simulink model "mcb_microchip_pmsm_foc_QDEC_Host_PIC32MK1024MCM"  (R2023b)
settings: Solver=FixedStepDiscrete  StartTime=0.0  StopTime=inf  RelTol=1e-3  EnableMultiTasking=on
values from neighbouring files (symbols this model uses):
  PU_System = mcb_SetPUSystem(pmsm,inverter)    [mcb_microchip_pmsm_foc_QDEC_PIC32MK1024MCF_data.m]
  Ts = T_pwm    (= 8.33333333333e-05)    [mcb_microchip_pmsm_foc_QDEC_PIC32MK1024MCF_data.m]
  Ts_SerialCom = 10*T_pwm    (= 0.000833333333333)    [mcb_microchip_pmsm_foc_QDEC_PIC32MK1024MCF_data.m]
libraries: simulink x6, instrumentseriallib x3
settings Model: Creator=The MathWorks, Inc.  LastModifiedBy=I69995
settings SolverCC: AlgebraicLoopSolver=TrustRegion
settings DataIOCC: LimitDataPoints=on  SaveFormat=Array  ReturnWorkspaceOutputs=off
settings OptimizationCC: LifeSpan=1  EfficientTunableParamExpr=on
settings DebuggingCC: MergeDetectMultiDrivingBlocksExec=none  SolverPrmCheckMsg=warning  ParameterPrecisionLossMsg=none  UnconnectedInputMsg=warning  UnconnectedOutputMsg=warning  UnconnectedLineMsg=warning  AllowSymbolicDim=off  PregeneratedLibrarySubsystemCodeDiagnostic=none  SFUnexpectedBacktrackingDiag=warning  SFNoUnconditionalDefaultTransitionDiag=warning  SFExecutionAtInitializationDiag=none  ArithmeticOperatorsInVariantConditions=warning
settings HardwareCC: ProdBitPerPointer=32  ProdLargestAtomicFloat=None  ProdIntDivRoundTo=Undefined  ProdEndianess=Unspecified  ProdWordSize=32  ProdHWDeviceType=32-bit Generic
settings ModelReferenceCC: EnableRefExpFcnMdlSchedulingChecks=on  PropagateSignalLabelsOutOfModel=off
settings SFSimCC: SimUseLocalCustomCode=off  MATLABDynamicMemAlloc=off
settings RTWCC: Description=Real-Time Workshop Embedded Coder  SystemTargetFile=ert.tlc  TemplateMakefile=ert_default_tmf  GenerateReport=on  RTWUseLocalCustomCode=off  IncludeHyperlinkInReport=on  LaunchReport=on  GenerateTraceInfo=on  GenerateTraceReport=on  GenerateTraceReportSl=on  GenerateTraceReportSf=on  GenerateTraceReportEml=on  DLArmComputeVersion=19.05
settings CodeAppCC: IgnoreCustomStorageClasses=off  StateflowObjectComments=on  InternalIdentifier=Classic
settings ERTTargetCC: MultiwordLength=2048  GenerateSampleERTMain=on  ERTCustomFileTemplate=example_file_process.tlc  ConvertIfToSwitch=off  SuppressUnreachableDefaultCases=off
settings ConfigComp: CovMetricSettings=dw  CovSaveCumulativeToWorkspaceVar=on  CovSaveSingleToWorkspaceVar=on  CovExternalEMLEnable=off  CovSFcnEnable=off

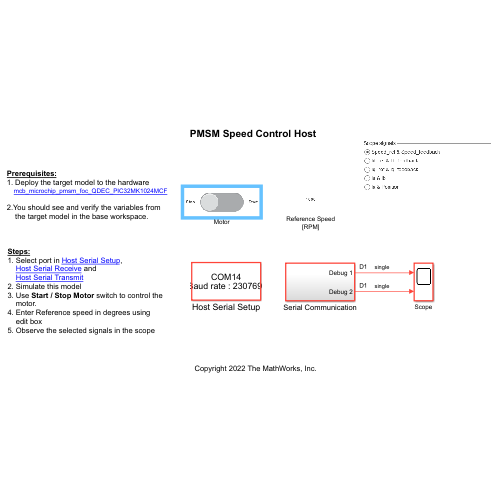
[thumbnail: Simulink's stored preview of the top-level diagram]
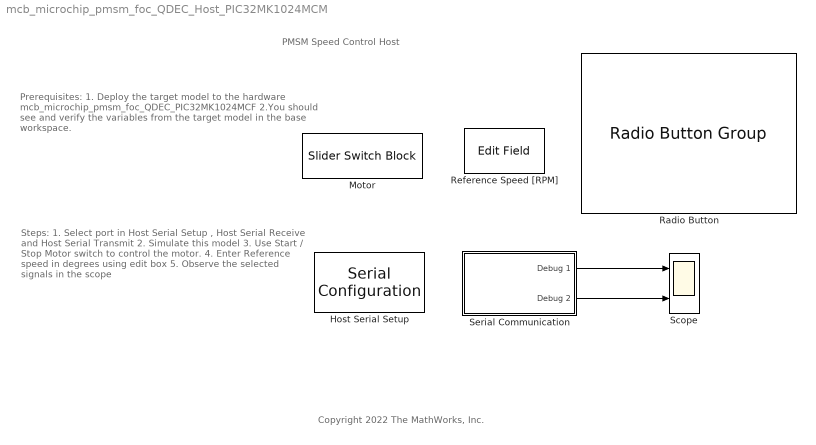
== system mcb_microchip_pmsm_foc_QDEC_Host_PIC32MK1024MCM ==
  note: PMSM Speed Control Host
  note: Copyright 2022 The MathWorks, Inc.
  note: Prerequisites:
      | 1. Deploy the target model to the hardware
      | mcb_microchip_pmsm_foc_QDEC_PIC32MK1024MCF
      |
      | 2.You should see and verify the variables from
      | the target model in the base workspace.
  note: Steps:
      | 1. Select port in Host Serial Setup ,
      | Host Serial Receive and
      | Host Serial Transmit
      | 2. Simulate this model
      | 3. Use Start / Stop Motor switch to control the
      | motor.
      | 4. Enter Reference speed in degrees using
      | edit box
      | 5. Observe the selected signals in the scope
  Host Serial Setup : instrumentseriallib/Serial Configuration  Priority=-99  PortSel=COM14  Port=COM14  ComPort=COM14  BaudRate=2307692  DataBits=8  Parity=none  StopBits=1  ByteOrder=little-endian  FlowControl=none  Timeout=2  SimulateUsing=Interpreted execution  BlockInModel=on  aMode=5
  Motor : SliderSwitchBlock  LabelPosition=Hide
      settings: Values={{'Stop', 'Start'}, [0 1]}
  Radio Button : RadioButtonGroup  LabelPosition=Hide  SelectedLabel=Speed_ref & Speed_feedback  ButtonGroupName=Scope signals
      settings: Values={{'Speed_ref & Speed_feedback', 'Id_ref & Id_feedback', 'Iq_ref & Iq_feedback', 'Ia & Ib', 'Ia & Position'}, [1 2 3 4 5]}
  Reference Speed [RPM] : EditField  LabelPosition=Hide  ShowInitialText=on  Alignment=Center
  Scope : Scope  NumInputPorts=2
  Serial Communication : Subsystem
  wires:
  Serial Communication/1(Debug 1) -> Scope/1
  Serial Communication/2(Debug 2) -> Scope/2

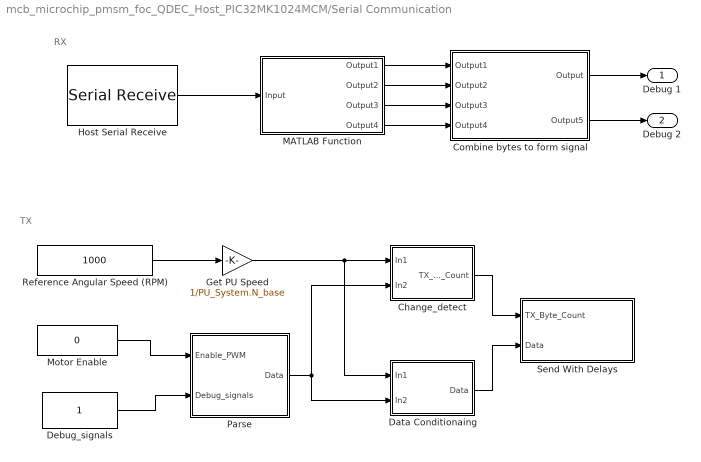
== system mcb_microchip_pmsm_foc_QDEC_Host_PIC32MK1024MCM/Serial Communication ==
  note: RX
  note: TX
  Change_detect : Subsystem
  Combine bytes to form signal : Subsystem
  Data Conditionaing : Subsystem  VariantControl=~isequal(dataType, 'single')
  Debug_signals : Constant  OutDataTypeStr=uint8  SampleTime=600 * Ts
  Get PU Speed : Gain  Gain=1/PU_System.N_base  OutDataTypeStr=fixdt(1,16,10)  RndMeth=Simplest
  Host Serial Receive : instrumentseriallib/Serial Receive  PortSel=COM14  Port=COM14  ComPort=COM14  DataType=uint8  SaveDataType=uint8  ToggleHeader=on  Header='S'  ToggleTerminator=on  Terminator=Custom terminator  CustomTerminator='E'  InputFormat=Row major  ToggleDataSize=on  DataSize=[60 4]  EnableBlockingMode=on  ActionDataUnavailable=Output last received value  ActionWhenDataUnavailable=Output last received value  CustomValue=15  SampleTime=60 * Ts_SerialCom  SimulateUsing=Interpreted execution  BlockInModel=on  aMode=5
  MATLAB Function : MATLAB Function  TreatAsAtomicUnit=on
  Motor Enable : Constant  Value=0  VectorParams1D=off  OutDataTypeStr=uint8  SampleTime=600 * Ts
  Parse : Subsystem
  Reference Angular Speed (RPM) : Constant  Value=1000  VectorParams1D=off  OutDataTypeStr=single  SampleTime=600 * Ts
  Send With Delays : Subsystem
  Debug 1 : Outport
  Debug 2 : Outport  Port=2
  wires:
  Host Serial Receive/1 -> MATLAB Function/1(Input)
  Combine bytes to form signal/1(Output) -> Debug 1/1
  Combine bytes to form signal/2(Output5) -> Debug 2/1
  Debug_signals/1 -> Parse/2(Debug_signals)
  Motor Enable/1 -> Parse/1(Enable_PWM)
  Parse/1(Data) -> Data Conditionaing/2(In2), Change_detect/2(In2)
  Reference Angular Speed (RPM)/1 -> Get PU Speed/1
  MATLAB Function/1(Output1) -> Combine bytes to form signal/1(Output1)
  MATLAB Function/2(Output2) -> Combine bytes to form signal/2(Output2)
  MATLAB Function/3(Output3) -> Combine bytes to form signal/3(Output3)
  MATLAB Function/4(Output4) -> Combine bytes to form signal/4(Output4)
  Change_detect/1(TX_Byte_Count) -> Send With Delays/1(TX_Byte_Count)
  Data Conditionaing/1(Data) -> Send With Delays/2(Data)
  Get PU Speed/1 -> Data Conditionaing/1(In1), Change_detect/1(In1)

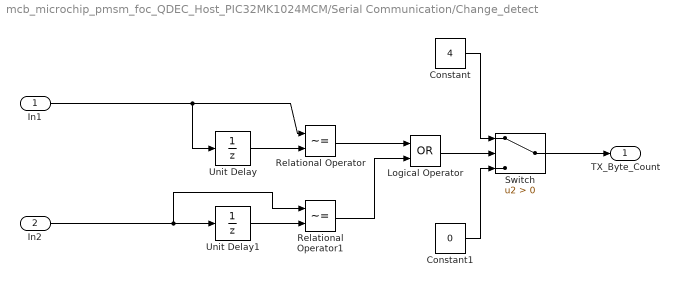
== system mcb_microchip_pmsm_foc_QDEC_Host_PIC32MK1024MCM/Serial Communication/Change_detect ==
  In1 : Inport
  In2 : Inport  Port=2
  Constant : Constant  Value=4  OutDataTypeStr=uint8
  Constant1 : Constant  Value=0  OutDataTypeStr=uint8
  Logical Operator : Logic  Operator=OR  AllPortsSameDT=off  OutDataTypeStr=boolean
  Relational Operator : RelationalOperator  Operator=~=  OutDataTypeStr=boolean  InputSameDT=off
  Relational Operator1 : RelationalOperator  Operator=~=  OutDataTypeStr=boolean  InputSameDT=off
  Switch : Switch  Criteria=u2 > Threshold  SaturateOnIntegerOverflow=off  InputSameDT=off
  Unit Delay : UnitDelay  InitialCondition=0.5  SampleTime=-1  HasFrameUpgradeWarning=on
  Unit Delay1 : UnitDelay  SampleTime=-1  HasFrameUpgradeWarning=on
  TX_Byte_Count : Outport  VectorParamsAs1DForOutWhenUnconnected=off
  wires:
  Relational Operator/1 -> Logical Operator/1
  In1/1 -> Relational Operator/1, Unit Delay/1
  Unit Delay/1 -> Relational Operator/2
  Unit Delay1/1 -> Relational Operator1/2
  Relational Operator1/1 -> Logical Operator/2
  In2/1 -> Unit Delay1/1, Relational Operator1/1
  Constant1/1 -> Switch/3
  Constant/1 -> Switch/1
  Logical Operator/1 -> Switch/2
  Switch/1 -> TX_Byte_Count/1

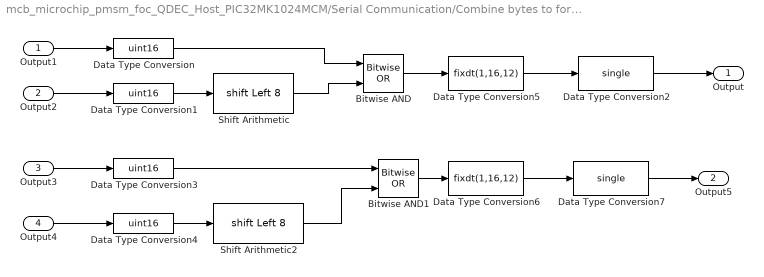
== system mcb_microchip_pmsm_foc_QDEC_Host_PIC32MK1024MCM/Serial Communication/Combine bytes to form signal ==
  Output1 : Inport
  Output2 : Inport  Port=2
  Output3 : Inport  Port=3
  Output4 : Inport  Port=4
  Bitwise AND : simulink/Logic and Bit Operations/Bitwise Operator  logicop=OR  UseBitMask=off  NumInputPorts=2  BitMask=bin2dec('11011001')  BitMaskRealWorld=Stored Integer
  Bitwise AND1 : simulink/Logic and Bit Operations/Bitwise Operator  logicop=OR  UseBitMask=off  NumInputPorts=2  BitMask=bin2dec('11011001')  BitMaskRealWorld=Stored Integer
  Data Type Conversion{,1,3..4} (4 alike) : DataTypeConversion  OutDataTypeStr=uint16  RndMeth=Simplest  SaturateOnIntegerOverflow=off
  Data Type Conversion2 : DataTypeConversion  OutDataTypeStr=single  RndMeth=Simplest  SaturateOnIntegerOverflow=off
  Data Type Conversion5 : DataTypeConversion  OutDataTypeStr=fixdt(1,16,12)  ConvertRealWorld=Stored Integer (SI)  RndMeth=Simplest  SaturateOnIntegerOverflow=off
  Data Type Conversion6 : DataTypeConversion  OutDataTypeStr=fixdt(1,16,12)  ConvertRealWorld=Stored Integer (SI)  RndMeth=Simplest  SaturateOnIntegerOverflow=off
  Data Type Conversion7 : DataTypeConversion  OutDataTypeStr=single  RndMeth=Simplest  SaturateOnIntegerOverflow=off
  Shift Arithmetic : ArithShift  BitShiftNumber=8  BitShiftDirection=Left
  Shift Arithmetic2 : ArithShift  BitShiftNumber=8  BitShiftDirection=Left
  Output : Outport
  Output5 : Outport  Port=2
  wires:
  Output1/1 -> Data Type Conversion/1
  Data Type Conversion5/1 -> Data Type Conversion2/1
  Output2/1 -> Data Type Conversion1/1
  Bitwise AND/1 -> Data Type Conversion5/1
  Data Type Conversion1/1 -> Shift Arithmetic/1
  Data Type Conversion/1 -> Bitwise AND/1
  Output3/1 -> Data Type Conversion3/1
  Output4/1 -> Data Type Conversion4/1
  Data Type Conversion4/1 -> Shift Arithmetic2/1
  Shift Arithmetic/1 -> Bitwise AND/2
  Bitwise AND1/1 -> Data Type Conversion6/1
  Data Type Conversion6/1 -> Data Type Conversion7/1
  Data Type Conversion3/1 -> Bitwise AND1/1
  Shift Arithmetic2/1 -> Bitwise AND1/2
  Data Type Conversion2/1 -> Output/1
  Data Type Conversion7/1 -> Output5/1

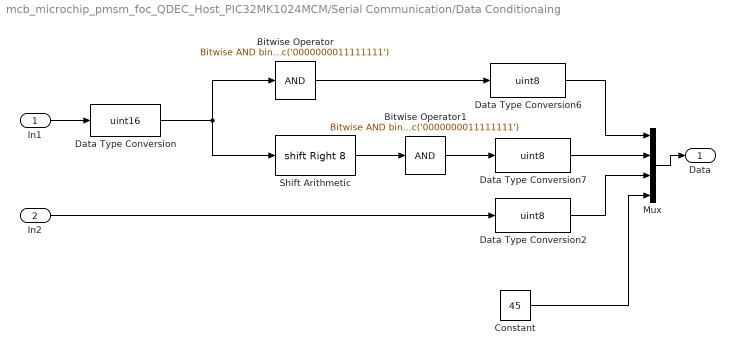
== system mcb_microchip_pmsm_foc_QDEC_Host_PIC32MK1024MCM/Serial Communication/Data Conditionaing ==
  In1 : Inport
  In2 : Inport  Port=2
  Bitwise Operator : simulink/Logic and Bit Operations/Bitwise Operator  logicop=AND  UseBitMask=on  BitMask=bin2dec('0000000011111111')  BitMaskRealWorld=Stored Integer
  Bitwise Operator1 : simulink/Logic and Bit Operations/Bitwise Operator  logicop=AND  UseBitMask=on  BitMask=bin2dec('0000000011111111')  BitMaskRealWorld=Stored Integer
  Constant : Constant  Value=45  OutDataTypeStr=uint8
  Data Type Conversion : DataTypeConversion  OutDataTypeStr=uint16  ConvertRealWorld=Stored Integer (SI)  RndMeth=Simplest  SaturateOnIntegerOverflow=off
  Data Type Conversion2 : DataTypeConversion  OutDataTypeStr=uint8  RndMeth=Simplest  SaturateOnIntegerOverflow=off
  Data Type Conversion6 : DataTypeConversion  OutDataTypeStr=uint8  RndMeth=Simplest  SaturateOnIntegerOverflow=off
  Data Type Conversion7 : DataTypeConversion  OutDataTypeStr=uint8  RndMeth=Simplest  SaturateOnIntegerOverflow=off
  Mux : Mux
  Shift Arithmetic : ArithShift  BitShiftNumber=8  BitShiftDirection=Right
  Data : Outport
  wires:
  Mux/1 -> Data/1
  Data Type Conversion6/1 -> Mux/1
  In1/1 -> Data Type Conversion/1
  Data Type Conversion/1 -> Shift Arithmetic/1, Bitwise Operator/1
  Bitwise Operator/1 -> Data Type Conversion6/1
  Shift Arithmetic/1 -> Bitwise Operator1/1
  Bitwise Operator1/1 -> Data Type Conversion7/1
  Data Type Conversion7/1 -> Mux/2
  Data Type Conversion2/1 -> Mux/3
  In2/1 -> Data Type Conversion2/1
  Constant/1 -> Mux/4

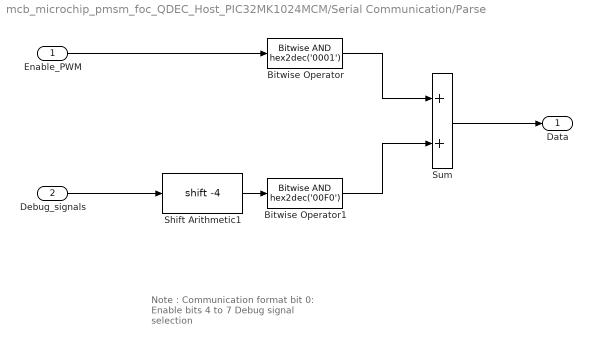
== system mcb_microchip_pmsm_foc_QDEC_Host_PIC32MK1024MCM/Serial Communication/Parse ==
  note: Note : Communication format
      | bit 0: Enable
      | bits 4 to 7 Debug signal selection
  Enable_PWM : Inport
  Debug_signals : Inport  Port=2
  Bitwise Operator : simulink/Logic and Bit Operations/Bitwise Operator  logicop=AND  UseBitMask=on  BitMask=hex2dec('0001')  BitMaskRealWorld=Stored Integer
  Bitwise Operator1 : simulink/Logic and Bit Operations/Bitwise Operator  logicop=AND  UseBitMask=on  BitMask=hex2dec('00F0')  BitMaskRealWorld=Stored Integer
  Shift Arithmetic1 : ArithShift  BitShiftNumber=-4
  Sum : Sum
  Data : Outport
  wires:
  Bitwise Operator1/1 -> Sum/2
  Enable_PWM/1 -> Bitwise Operator/1
  Shift Arithmetic1/1 -> Bitwise Operator1/1
  Sum/1 -> Data/1
  Debug_signals/1 -> Shift Arithmetic1/1
  Bitwise Operator/1 -> Sum/1

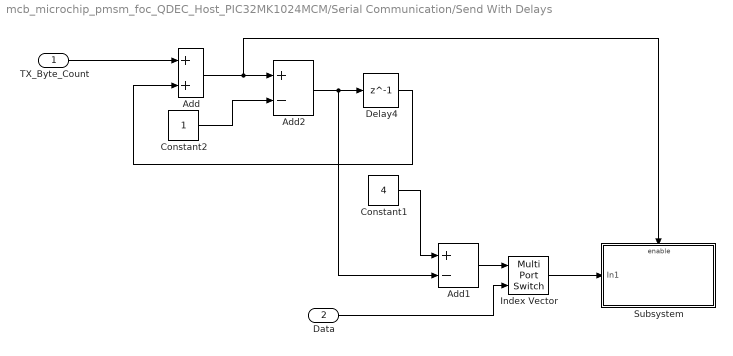
== system mcb_microchip_pmsm_foc_QDEC_Host_PIC32MK1024MCM/Serial Communication/Send With Delays ==
  TX_Byte_Count : Inport
  Data : Inport  Port=2
  Add : Sum  SaturateOnIntegerOverflow=on
  Add1 : Sum  Inputs=+-  SaturateOnIntegerOverflow=on
  Add2 : Sum  Inputs=+-  SaturateOnIntegerOverflow=on
  Constant1 : Constant  Value=4  OutDataTypeStr=uint8
  Constant2 : Constant  OutDataTypeStr=uint8
  Delay4 : Delay  DelayLength=1
  Index Vector : MultiPortSwitch  Inputs=1  SaturateOnIntegerOverflow=off  InputSameDT=off
  Subsystem : Subsystem
  wires:
  Data/1 -> Index Vector/2
  TX_Byte_Count/1 -> Add/1
  Add/1 -> Subsystem/Enable, Add2/1
  Delay4/1 -> Add/2
  Add1/1 -> Index Vector/1
  Constant1/1 -> Add1/1
  Index Vector/1 -> Subsystem/1(In1)
  Add2/1 -> Add1/2, Delay4/1
  Constant2/1 -> Add2/2

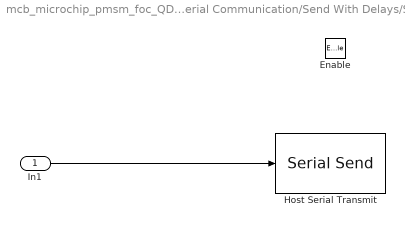
== system mcb_microchip_pmsm_foc_QDEC_Host_PIC32MK1024MCM/Serial Communication/Send With Delays/Subsystem ==
  In1 : Inport
  Enable : EnablePort
  Host Serial Transmit : instrumentseriallib/Serial Send  PortSel=COM14  Port=COM14  ComPort=COM14  Header=[]  Terminator=<none>  CustomTerminator=[]  EnableBlockingMode=off  SimulateUsing=Interpreted execution  BlockInModel=on  aMode=5
  wires:
  In1/1 -> Host Serial Transmit/1

== matlab function mcb_microchip_pmsm_foc_QDEC_Host_PIC32MK1024MCM/Serial Communication/MATLAB Function ==
  data: Output1 output; Output2 output; Input input; Output3 output; Output4 output
function [ Output1, Output2, Output3, Output4] = unBuf(Input)

Output1= Input(:, 1);
Output2 = Input(:, 2);
Output3 = Input(:, 3);
Output4 = Input(:, 4);

end
